simulink model "CollisionAvoidance_Demo"  (R2022a)
settings: Solver=FixedStepDiscrete  StartTime=0.0  StopTime=10.0  RelTol=1e-3
model workspace (MAT data in the model file):
  EgoCarParams.v0_ego = 4.55
  EgoCarParams.x0_ego = 8.3
  EgoCarParams.y0_ego = 0
  EgoCarParams.yaw0_ego = 0
  EgoCarParams.m = 1575
  EgoCarParams.Iz = 2875
  EgoCarParams.lf = 1.2
  EgoCarParams.lr = 1.6
  EgoCarParams.Cf = 19000
  EgoCarParams.Cr = 33000
  EgoCarParams.tau1 = 0.5
  EgoCarParams.tau2 = 0.07
libraries: dspindex x6, drivingscenarioandsensors x1
settings Model: Creator=Jim T  LastModifiedBy=11064

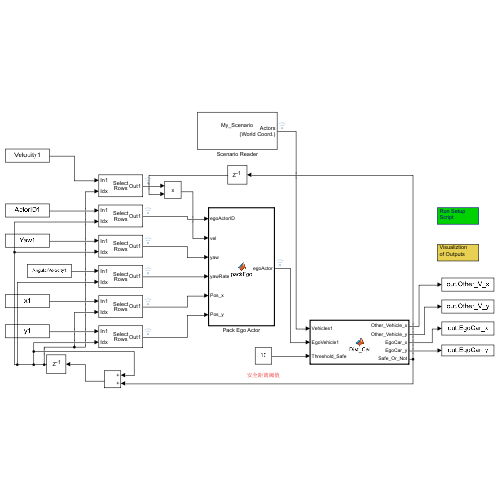
[thumbnail: Simulink's stored preview of the top-level diagram]
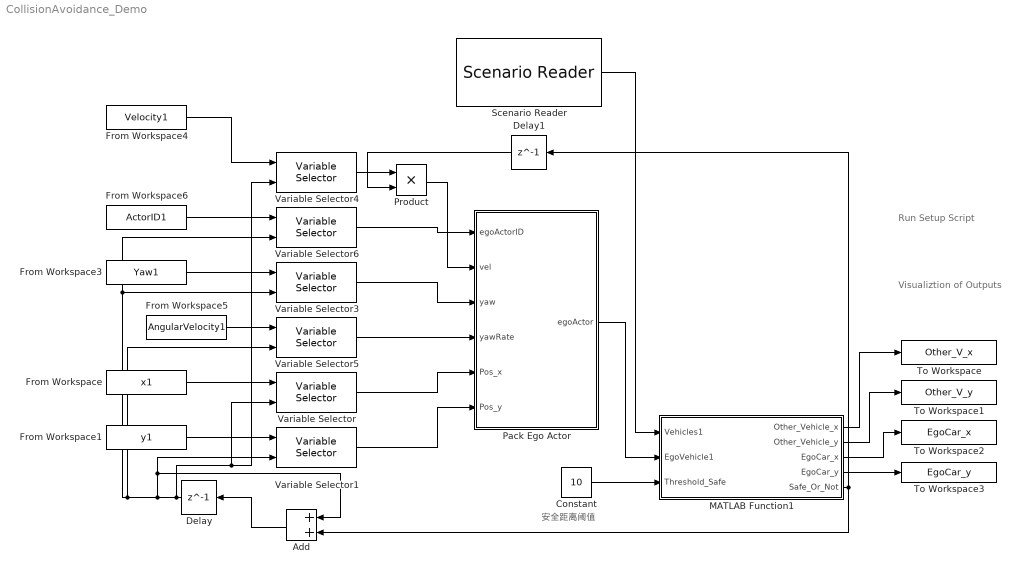
== system CollisionAvoidance_Demo ==
  note: Run Setup
      | Script
  note: 安全距离阈值
  note: Visualiztion
      | of Outputs
  Add : Sum
  Constant : Constant  Value=10
  Delay : Delay  DelayLength=1  InitialCondition=0
  Delay1 : Delay  DelayLength=1  InitialCondition=0
  From Workspace : FromWorkspace  VariableName=x1
  From Workspace1 : FromWorkspace  VariableName=y1
  From Workspace3 : FromWorkspace  VariableName=Yaw1
  From Workspace4 : FromWorkspace  VariableName=Velocity1
  From Workspace5 : FromWorkspace  VariableName=AngularVelocity1
  From Workspace6 : FromWorkspace  VariableName=ActorID1
  MATLAB Function1 : MATLAB Function  TreatAsAtomicUnit=on
  Pack Ego Actor : MATLAB Function  TreatAsAtomicUnit=on
  Product : Product
  Scenario Reader : drivingscenarioandsensors/Scenario Reader  ScenarioSource=From file  ScenarioFileName=My_Scenario.mat  ScenarioVariableName=scenario  OutputCoordinateSystem=World coordinates  EgoVehicleSource=Scenario  EgoVehicleActorID=1  OrientVehiclesOnRoad=off  OutputEgoVehiclePose=on  OutputEgoVehicleState=off  SampleTime=0.1  LaneBoundaryOutput=None  LaneBoundaryDistance=0:0.5:9.5  LaneBoundaryLocation=Center of lane markings  BusNameSource=Auto  BusName=BusActors  BusNumActorsSource=Scenario  BusNumActors=100  BusName2Source=Auto  BusName2=BusLaneBoundaries  BusNumLaneBoundariesSource=Scenario  BusNumLaneBoundaries=10  BusName3Source=Auto  BusName3=BusEgoActor  BusName4Source=Auto  BusName4=BusEgoState  ShowCoordinateLabels=on  SimulateUsing=Interpreted execution
  To Workspace : ToWorkspace  VariableName=Other_V_x  SampleTime=-1
      settings: Save2DSignal=2-D array (concatenate along first dimension)
  To Workspace1 : ToWorkspace  VariableName=Other_V_y  SampleTime=-1
      settings: Save2DSignal=2-D array (concatenate along first dimension)
  To Workspace2 : ToWorkspace  VariableName=EgoCar_x  SampleTime=-1
      settings: Save2DSignal=2-D array (concatenate along first dimension)
  To Workspace3 : ToWorkspace  VariableName=EgoCar_y  SampleTime=-1
      settings: Save2DSignal=2-D array (concatenate along first dimension)
  Variable Selector{,1,3..6} (6 alike) : dspindex/Variable Selector  NumInputs=1  rowsOrCols=Rows  IdxMode=Variable  Elements=[1 3]  ZerOneIdxMode=One-based  errmode=Clip Index  FillMode=on  FillValues=0
  wires:
  MATLAB Function1/2(Other_Vehicle_y) -> To Workspace1/1
  MATLAB Function1/3(EgoCar_x) -> To Workspace2/1
  MATLAB Function1/1(Other_Vehicle_x) -> To Workspace/1
  MATLAB Function1/4(EgoCar_y) -> To Workspace3/1
  Constant/1 -> MATLAB Function1/3(Threshold_Safe)
  Product/1 -> Pack Ego Actor/2(vel)
  From Workspace6/1 -> Variable Selector6/1
  Delay1/1 -> Product/2
  Variable Selector4/1 -> Product/1
  Pack Ego Actor/1(egoActor) -> MATLAB Function1/2(EgoVehicle1)
  Variable Selector1/1 -> Pack Ego Actor/6(Pos_y)
  Variable Selector/1 -> Pack Ego Actor/5(Pos_x)
  Variable Selector6/1 -> Pack Ego Actor/1(egoActorID)
  Variable Selector5/1 -> Pack Ego Actor/4(yawRate)
  From Workspace5/1 -> Variable Selector5/1
  From Workspace3/1 -> Variable Selector3/1
  From Workspace4/1 -> Variable Selector4/1
  Variable Selector3/1 -> Pack Ego Actor/3(yaw)
  From Workspace/1 -> Variable Selector/1
  Add/1 -> Delay/1
  From Workspace1/1 -> Variable Selector1/1
  Scenario Reader/1 -> MATLAB Function1/1(Vehicles1)
  Delay/1 -> Variable Selector6/2, Variable Selector3/2, Variable Selector5/2, Variable Selector1/2, Add/1, Variable Selector4/2, Variable Selector/2
  MATLAB Function1/5(Safe_Or_Not) -> Delay1/1, Add/2

== matlab function CollisionAvoidance_Demo/MATLAB Function1 ==
  data: Other_Vehicle_x output; Other_Vehicle_y output; EgoCar_x output; EgoCar_y output; Vehicles1 input; EgoVehicle1 input; Safe_Or_Not output; Threshold_Safe input
function [Other_Vehicle_x,Other_Vehicle_y,EgoCar_x,EgoCar_y ,Safe_Or_Not] = Dist_Cal (Vehicles1, EgoVehicle1,Threshold_Safe)

Other_Vehicle_x=Vehicles1.Actors(2).Position(:,1);
Other_Vehicle_y=Vehicles1.Actors(2).Position(:,2);

EgoCar_x=EgoVehicle1.Position(:,1);
EgoCar_y=EgoVehicle1.Position(:,2);

Distance_1=sqrt((Other_Vehicle_x-EgoCar_x)^2+(Other_Vehicle_y-EgoCar_y)^2);


if Distance_1 > Threshold_Safe

    Safe_Or_Not=1;

else 

    Safe_Or_Not=0;

end

== matlab function CollisionAvoidance_Demo/Pack Ego Actor ==
  data: egoActorID input; vel input; yaw input; yawRate input; Pos_x input; egoActor output Bus: BusActorsActors size=1; Pos_y input
function egoActor = packEgo(egoActorID,vel,yaw,yawRate,Pos_x,Pos_y)
% Pack ego information into a single ego actor bus
%
% Imoprtant note:
% Output is a bus of type BusActorsActors. This is the same bus used by the
% Scenario Reader to output an individual actor. If you change the
% output bus name of Scenario Reader, change the output bus name here
% as well by clicking on 'Edit Data' in the menu above.

egoActor = struct(...
    'ActorID',egoActorID,...
    'Position', [Pos_x Pos_y 0], ...
    'Velocity', [vel(1) vel(2) 0], ...
    'Roll', 0, ...
    'Pitch', 0, ...
    'Yaw', yaw, ...
    'AngularVelocity',yawRate);
%  'AngularVelocity', [0 0 yawRate]);
